simulink model "dabClosedLoop"  (R2017a)
settings: Solver=ode45  StartTime=0.0  StopTime=1  MaxStep=1e-4  RelTol=1e-3
libraries: powerlib x23, simulink x1
settings Model: Creator=Lenovo  LastModifiedBy=Lenovo

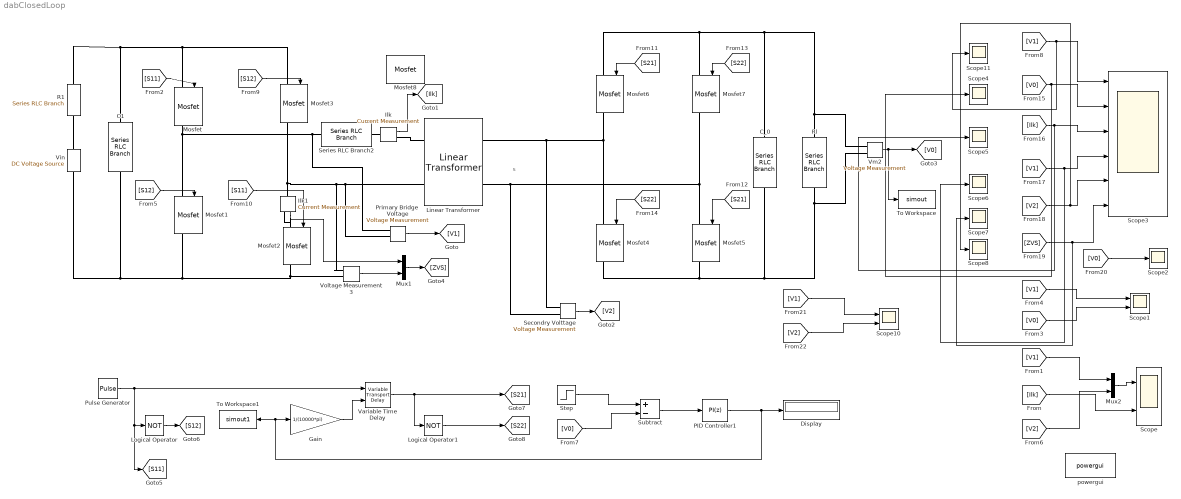
== system dabClosedLoop ==
  note: s
  C1 : powerlib/Elements/Series RLC Branch  LConnTagsString=__new0  RConnTagsString=__new0  BranchType=C  Resistance=0.4  Inductance=800e-6  SetiL0=off  InitialCurrent=0  Capacitance=1600e-6  Setx0=off  InitialVoltage=0  Measurements=None
  C_0 : powerlib/Elements/Series RLC Branch  LConnTagsString=__new0  RConnTagsString=__new0  BranchType=RC  Resistance=0.0001  Inductance=1e-3  SetiL0=off  InitialCurrent=0  Capacitance=2600e-6  Setx0=off  InitialVoltage=0  Measurements=None
  Display : Display
  Gain : Gain  Gain=1/(10000*pi)
  Ilk : powerlib/Measurements/Current Measurement  PhasorSimulation=off  OutputType=Complex  PSBequivalent=0
  Ilk1 : powerlib/Measurements/Current Measurement  PhasorSimulation=off  OutputType=Complex  PSBequivalent=0
  Linear Transformer : powerlib/Elements/Linear Transformer  UNITS=SI  NominalPower=[3500e6 10000*pi]  winding1=[500 0 0]  winding2=[250 0 0]  ThreeWindings=off  winding3=[3.15e+05 0.7938 0.084225]  RmLm=[1.0804e+06 2866]  Measurements=None  DataType=on
  Logical Operator : Logic  Operator=NOT  AllPortsSameDT=off  OutDataTypeStr=boolean
  Logical Operator1 : Logic  Operator=NOT  AllPortsSameDT=off  OutDataTypeStr=boolean
  Mosfet : powerlib/Power Electronics/Mosfet  Ron=0.1  Lon=0  Rd=0.07  Vfd=0  IC=0  Rs=1e5  Cs=inf  Measurements=on
  Mosfet1 : powerlib/Power Electronics/Mosfet  Ron=0.1  Lon=0  Rd=0.07  Vfd=0  IC=0  Rs=1e5  Cs=inf  Measurements=on
  Mosfet2 : powerlib/Power Electronics/Mosfet  Ron=0.1  Lon=0  Rd=0.01  Vfd=0  IC=0  Rs=1e5  Cs=inf  Measurements=on
  Mosfet3 : powerlib/Power Electronics/Mosfet  Ron=0.1  Lon=0  Rd=0.07  Vfd=0  IC=0  Rs=1e5  Cs=inf  Measurements=on
  Mosfet{4..7} (4 alike) : powerlib/Power Electronics/Mosfet  Ron=0.01  Lon=0  Rd=0.01  Vfd=0  IC=0  Rs=1e5  Cs=inf  Measurements=on
  Mosfet8 : powerlib/Power Electronics/Mosfet  Ron=0.1  Lon=0  Rd=0.01  Vfd=0  IC=0  Rs=1e5  Cs=inf  Measurements=on
  Mux1 : Mux  Inputs=2
  Mux2 : Mux  Inputs=2
  PID Controller1 : simulink/Continuous/PID Controller  Controller=PI  TimeDomain=Discrete-time  SampleTime=1e-6  IntegratorMethod=Forward Euler  FilterMethod=Forward Euler  Form=Parallel  UseFilter=on  ControllerParametersSource=internal  P=0.029  I=0.155  D=0  N=100  InitialConditionSource=internal  InitialConditionForIntegrator=0  InitialConditionForFilter=0  ExternalReset=none  LimitOutput=on  UpperSaturationLimit=1  LowerSaturationLimit=-1  LinearizeAsGain=on  AntiWindupMode=none  Kb=1  TrackingMode=off  Kt=1  PParamMin=[]  PParamMax=[]  IParamMin=[]  IParamMax=[]  DParamMin=[]  DParamMax=[]  NParamMin=[]  NParamMax=[]  KbParamMin=[]  KbParamMax=[]  KtParamMin=[]  KtParamMax=[]  POutMin=[]  POutMax=[]  IOutMin=[]  IOutMax=[]  DOutMin=[]  DOutMax=[]  NOutMin=[]  NOutMax=[]  KbOutMin=[]  KbOutMax=[]  KtOutMin=[]  KtOutMax=[]  IntegratorOutMin=[]  IntegratorOutMax=[]  FilterOutMin=[]  FilterOutMax=[]  SumOutMin=[]  SumOutMax=[]  SumI1OutMin=[]  SumI1OutMax=[]  SumI2OutMin=[]  SumI2OutMax=[]  SumI3OutMin=[]  SumI3OutMax=[]  SumDOutMin=[]  SumDOutMax=[]  SaturationOutMin=[]  SaturationOutMax=[]  IntegratorContinuousStateAttributes=''  IntegratorStateMustResolveToSignalObject=off  IntegratorRTWStateStorageClass=Auto  FilterContinuousStateAttributes=''  FilterStateMustResolveToSignalObject=off  FilterRTWStateStorageClass=Auto  DifferentiatorICPrevScaledInput=0  DifferentiatorOutMin=[]  DifferentiatorOutMax=[]  InitialConditionSetting=State (most efficient)
  Primary Bridge  Voltage : powerlib/Measurements/Voltage Measurement  PhasorSimulation=off  OutputType=Complex  PSBequivalent=0
  Pulse Generator : DiscretePulseGenerator  PulseType=Time based  Period=1/(10000)  PulseWidth=50
  R1 : powerlib/Elements/Series RLC Branch  LConnTagsString=__new0  RConnTagsString=__new0  BranchType=R  Resistance=1  Inductance=800e-6  SetiL0=off  InitialCurrent=0  Capacitance=1550e-6  Setx0=off  InitialVoltage=0  Measurements=None
  Rl : powerlib/Elements/Series RLC Branch  LConnTagsString=__new0  RConnTagsString=__new0  BranchType=R  Resistance=35  Inductance=1e-3  SetiL0=off  InitialCurrent=0  Capacitance=1e-6  Setx0=off  InitialVoltage=0  Measurements=None
  Scope : Scope  NumInputPorts=2
  Scope1 : Scope  NumInputPorts=2
  Scope10 : Scope  NumInputPorts=2
  Scope{2,4..8,11} (7 alike) : Scope
  Scope3 : Scope  NumInputPorts=6
  Secondry Volttage : powerlib/Measurements/Voltage Measurement  PhasorSimulation=off  OutputType=Complex  PSBequivalent=0
  Series RLC Branch2 : powerlib/Elements/Series RLC Branch  LConnTagsString=__new0  RConnTagsString=__new0  BranchType=RL  Resistance=0.007  Inductance=900e-6  SetiL0=off  InitialCurrent=0  Capacitance=1e-6  Setx0=off  InitialVoltage=0  Measurements=None
  Step : Step  Time=0.5  Before=60  After=90  SampleTime=0
  Subtract : Sum  Inputs=+-
  To Workspace : ToWorkspace  VariableName=simout  SampleTime=1/10000
  To Workspace1 : ToWorkspace  VariableName=simout1  SampleTime=1/10000
  Variable Time Delay : VariableTransportDelay  MaximumDelay=10
  Vin : powerlib/Electrical Sources/DC Voltage Source  Amplitude=126  Measurements=None
  Vm2 : powerlib/Measurements/Voltage Measurement  PhasorSimulation=off  OutputType=Complex  PSBequivalent=0
  Voltage Measurement3 : powerlib/Measurements/Voltage Measurement  PhasorSimulation=off  OutputType=Complex  PSBequivalent=0
  powergui : powerlib/powergui  Priority=1  SimulationMode=Continuous  SampleTime=50e-6  frequency=60  Iterations=50  frequencyindice=0  Pbase=100e6  ErrMax=1e-4  UnitsV=kV  UnitsW=MW  buscounter=0  FunctionMessages=off  echomessages=off  EnableUseOfTLC=off  CurrentSourceSwitches=off  DisableSnubberDevices=off  DisableRonSwitches=off  DisableVfSwitches=off  DisplayEquations=off  SolverType=Tustin/Backward Euler (TBE)  Interpol=off  ExternalGateDelay=off  methode=off  Ts=100  x0status=blocks  SPID=on  SwTol=0  HookPort=off  RestoreLinks=warning  ResistiveCurrentMeasurement=off  Frange=[0:2:500]  Ylog=off  Xlog=on  ShowGrid=off  save=off  variable=ZData  structure=0  ZoomFFT=off  StartTime=0.0  cycles=1  DisplayStyle=1  fundamental=60  FreqAxis=off  MaxFrequency=1000  frequencyindicesteady=1  RmsSteady=1  display=off
  wires:
  [V0] -> Subtract/2
  Secondry Volttage/1 -> [V2]
  Subtract/1 -> PID Controller1/1
  [ZVS] -> Scope7/1, Scope3/6
  [S12] -> Mosfet1/1
  Mux1/1 -> [ZVS]
  [V1] -> Scope6/1, Scope3/4
  [S11] -> Mosfet2/1
  [V2] -> Scope8/1, Scope3/5
  Variable Time Delay/1 -> Logical Operator1/1, [S21]
  [V1] -> Scope11/1, Scope3/1
  Ilk/1 -> [Ilk]
  [V0] -> Scope4/1, Scope3/2
  [Ilk] -> Scope5/1, Scope3/3
  [S21] -> Mosfet5/1
  [S22] -> Mosfet4/1
  Logical Operator1/1 -> [S22]
  [S11] -> Mosfet/1
  [S22] -> Mosfet7/1
  Pulse Generator/1 -> Logical Operator/1, [S11], Variable Time Delay/1
  Primary Bridge  Voltage/1 -> [V1]
  Step/1 -> Subtract/1
  Gain/1 -> Variable Time Delay/2
  [S21] -> Mosfet6/1
  [V0] -> Scope1/2
  [S12] -> Mosfet3/1
  Ilk1/1 -> Mux1/1
  Logical Operator/1 -> [S12]
  PID Controller1/1 -> To Workspace1/1, Gain/1, Display/1
  Voltage Measurement3/1 -> Mux1/2
  [V1] -> Scope1/1
  Vm2/1 -> To Workspace/1, [V0]
  [V1] -> Mux2/1
  Mux2/1 -> Scope/1
  [V2] -> Mux2/2
  [Ilk] -> Scope/2
  [V0] -> Scope2/1
  [V1] -> Scope10/1
  [V2] -> Scope10/2
  connections:
  Primary Bridge  Voltage/LConn1 -- Mosfet1/LConn1 -- Mosfet/RConn1 -- Series RLC Branch2/LConn1
  Mosfet2/RConn1 -- C1/RConn1 -- Vin/LConn1 -- Mosfet1/RConn1 -- Voltage Measurement3/LConn2
  Mosfet5/LConn1 -- Mosfet7/RConn1 -- Linear Transformer/RConn2 -- Secondry Volttage/LConn2
  Rl/RConn1 -- C_0/RConn1 -- Mosfet5/RConn1 -- Mosfet4/RConn1 -- Vm2/LConn2
  Linear Transformer/RConn1 -- Mosfet4/LConn1 -- Mosfet6/RConn1 -- Secondry Volttage/LConn1
  Mosfet7/LConn1 -- C_0/LConn1 -- Rl/LConn1 -- Vm2/LConn1 -- Mosfet6/LConn1
  Mosfet/LConn1 -- R1/LConn1 -- C1/LConn1 -- Mosfet3/LConn1
  Linear Transformer/LConn2 -- Primary Bridge  Voltage/LConn2 -- Ilk1/LConn1 -- Mosfet3/RConn1 -- Voltage Measurement3/LConn1
  Ilk/LConn1 -- Series RLC Branch2/RConn1
  Linear Transformer/LConn1 -- Ilk/RConn1
  Mosfet2/LConn1 -- Ilk1/RConn1
  Vin/RConn1 -- R1/RConn1
